simulink subsystem "V5_SUB_DC_DC_Wandler"  (R2022b)
settings: Solver=VariableStepAuto  StartTime=0.0  StopTime=10.0  RelTol=1e-3
undefined symbols (not defined in the file or in its folder): C, L, R_L, R_Last
settings Model: Creator=JSCHB  LastModifiedBy=janbe

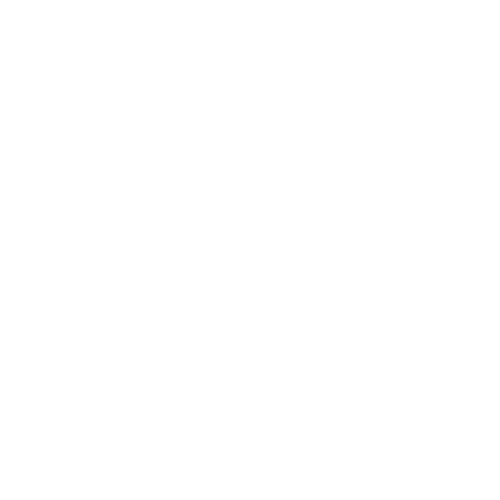
[thumbnail: Simulink's stored preview of the top-level diagram]
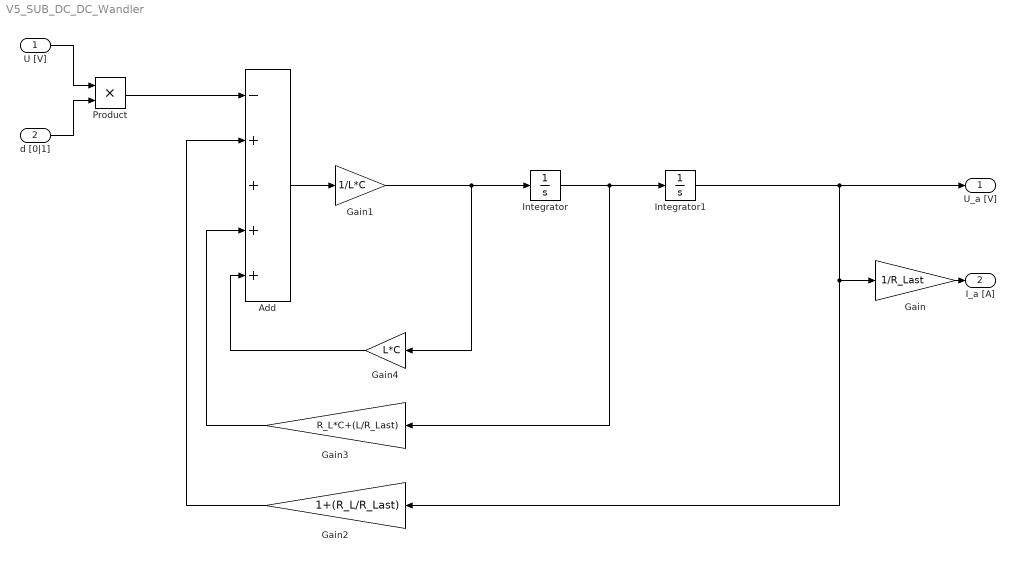
== system V5_SUB_DC_DC_Wandler ==
  U [V] : Inport
  d [0|1] : Inport  Port=2
  Add : Sum  Inputs=-++++
  Gain : Gain  Gain=1/R_Last
  Gain1 : Gain  Gain=1/L*C
  Gain2 : Gain  Gain=1+(R_L/R_Last)
  Gain3 : Gain  Gain=R_L*C+(L/R_Last)
  Gain4 : Gain  Gain=L*C
  Integrator : Integrator
  Integrator1 : Integrator
  Product : Product
  U_a [V] : Outport
  I_a [A] : Outport  Port=2
  wires:
  Gain2/1 -> Add/2
  Gain4/1 -> Add/5
  Gain3/1 -> Add/4
  Integrator/1 -> Integrator1/1, Gain3/1
  Integrator1/1 -> U_a [V]/1, Gain/1, Gain2/1
  Add/1 -> Gain1/1
  Gain1/1 -> Integrator/1, Gain4/1
  Product/1 -> Add/1
  d [0|1]/1 -> Product/2
  U [V]/1 -> Product/1
  Gain/1 -> I_a [A]/1
